simulink model "momentumBasedFlight"  (Simulink 10.3)
settings: Solver=FixedStepAuto  StartTime=0.0  StopTime=Config.simulationTime  FixedStep=Config.tStep  RelTol=1e-3
InitFcn:
  | cd(fileparts(which(bdroot)));
  | initMomentumBasedFlight;
StopFcn:
  | cd(fileparts(which(bdroot)));
  | stopMomentumBasedFlight;
undefined symbols (not defined in the file or in its folder): biasVectorConstraint_feet, Config, confVisualizer, ConstraintMatrix_feet, DiscIntNeverNeededParam, jets_config
undefined symbols (not defined in the file): Frames
libraries: WBToolboxLibrary x25, momentum_flight_control_sublib x2, thrust_estimation_sublib x1, jets_control x1, iDynVisualizer x1
(part 3 of 3)

== matlab function FLIGHT CONTROLLER (CORE) V2.5 - AERO/Flight Controller RAL-HUMANOIDS V3.0 - AERODYNAMICS/Joint Torque Control for Flying/torqueControlFCN ==
  data: M input double; h input double; J_jets input double; J_LFoot input double; J_RFoot input double; JDot_LFoot_nu input double; JDot_RFoot_nu input double; J_com input double; w_H_LFoot input double; w_H_RFoot input double; matrixOfJetsAxes input double; ConstraintsMatrix_feet input double; biasVectorConstraint_feet input double; jetsIntensities input double; stateVel input double; jointVel_star input double; contactForces_star input double; KI_torqueControl input double; KP_torqueControl input double; feetContactIsActive input double; activateEqConstrTorqueControl input double; robotIsLanded input double; jointPos_err input double; aerodynamic_force input double; Hessian output double; Config parameter double; gradient output double; ConstraintMatrix_inequality output double; biasVectorConstraint_inequality output double; jointVel_err output double
function [Hessian, gradient, ConstraintMatrix_inequality, biasVectorConstraint_inequality, jointVel_err] =  ... 
             flightTorqueControlFCN(M, h, J_jets, J_LFoot, J_RFoot, JDot_LFoot_nu, JDot_RFoot_nu, J_com, w_H_LFoot, w_H_RFoot, matrixOfJetsAxes, ...
                                    ConstraintsMatrix_feet, biasVectorConstraint_feet, jetsIntensities, stateVel, jointVel_star, contactForces_star, ...
                                    KI_torqueControl, KP_torqueControl, feetContactIsActive, activateEqConstrTorqueControl, robotIsLanded, jointPos_err, aerodynamic_force, Config)
                                      
    [Hessian, gradient, ConstraintMatrix_inequality, biasVectorConstraint_inequality, jointVel_err] =  ... 
             flightTorqueControl(M, h, J_jets, J_LFoot, J_RFoot, JDot_LFoot_nu, JDot_RFoot_nu, J_com, w_H_LFoot, w_H_RFoot, matrixOfJetsAxes, ...
                                 ConstraintsMatrix_feet, biasVectorConstraint_feet, jetsIntensities, stateVel, jointVel_star, contactForces_star, ...
                                 KI_torqueControl, KP_torqueControl, feetContactIsActive, activateEqConstrTorqueControl, robotIsLanded, jointPos_err, aerodynamic_force, Config);           
end

== matlab function FLIGHT CONTROLLER (CORE) V2.5 - AERO/Flight State Machine/Compute Gains And References/Trajectory Generator/Detect Robot Movement Request From Joystick ==
  data: joyAxes input double; moveFront output double; moveLateral output double; moveUpDown output double; rotateRoll output double; rotatePitch output double; joyButtons input double; rotateYaw output double; turbo_mode output double; goLandingPos output double
function [moveFront,moveLateral,moveUpDown,rotateRoll,rotatePitch,rotateYaw,turbo_mode,goLandingPos] = detectMovementsFromJoystickFCN(joyAxes,joyButtons)

    [moveFront,moveLateral,moveUpDown,rotateRoll,rotatePitch,rotateYaw,turbo_mode,goLandingPos] = iRonCubLib.detectMovementsFromJoystick(joyAxes,joyButtons);
end

== matlab function FLIGHT CONTROLLER (CORE) V2.5 - AERO/Flight State Machine/Take Off//Landing State Detector/MATLAB Function ==
  data: wrench_l input double; feetContactIsActive output double; wrench_r input double; Config parameter double; robotIsLanded output double; oneFootIsInContact output double
function [feetContactIsActive, robotIsLanded, oneFootIsInContact] = feetContactActivationFCN(wrench_l, wrench_r, Config)

    [feetContactIsActive, robotIsLanded, oneFootIsInContact] = iRonCubLib.feetContactActivation(wrench_l, wrench_r, Config);
end

== matlab function FLIGHT CONTROLLER (CORE) V2.5 - AERO/Flight Controller RAL-HUMANOIDS V3.0 - AERODYNAMICS/Momentum Control for Flying/Momentum Control/Flying Controller Momentum FCN  ==
  data: jointPos input double; w_baseTwist input double; jetsIntensities input double; J_jets input double; J_CoM input double; J_LFoot input double; J_RFoot input double; posCoM input double; w_R_b input double; w_H_LFoot input double; w_H_RFoot input double; matrixOfJetsAxes input double; matrixOfJetsArms input double; w_I_c input double; L input double; M input double; CMM input double; pos_vel_acc_jerk_CoM_des input double; rot_vel_acc_jerk_base_des input double size=[3,6]; jointPos_des input double; KP_momentum input double; KD_momentum input double; KP_postural input double; feetContactIsActive input double; decreaseMaxFootVerticalForce input double; increaseMinFootVerticalForce input double; robotIsLanded input double; HessianMatrixQP output double; gVectorQP output double; lowerBoundQP output double; upperBoundQP output double; L_des output double; LDot_estimated output double; verifyAngMomAndInertia output double; contactForces_hat input double; aerodynamic_force input double; Config parameter double
function [HessianMatrixQP, gVectorQP, lowerBoundQP, upperBoundQP, L_des, LDot_estimated, verifyAngMomAndInertia] = ...
             flightMomentumControlFCN(jointPos, w_baseTwist, jetsIntensities, J_jets, J_CoM, J_LFoot, J_RFoot, posCoM, w_R_b, w_H_LFoot, ...
                                      w_H_RFoot, matrixOfJetsAxes, matrixOfJetsArms, w_I_c, L, M, CMM, pos_vel_acc_jerk_CoM_des, ....
                                      rot_vel_acc_jerk_base_des, jointPos_des, KP_momentum, KD_momentum, KP_postural, feetContactIsActive, ...
                                      decreaseMaxFootVerticalForce, increaseMinFootVerticalForce, robotIsLanded, contactForces_hat, aerodynamic_force, Config)
                               
    [HessianMatrixQP, gVectorQP, lowerBoundQP, upperBoundQP, L_des, LDot_estimated, verifyAngMomAndInertia] = ...
             flightMomentumControl(jointPos, w_baseTwist, jetsIntensities, J_jets, J_CoM, J_LFoot, J_RFoot, posCoM, w_R_b, w_H_LFoot, ...
                                   w_H_RFoot, matrixOfJetsAxes, matrixOfJetsArms, w_I_c, L, M, CMM, pos_vel_acc_jerk_CoM_des, ....
                                   rot_vel_acc_jerk_base_des, jointPos_des, KP_momentum, KD_momentum, KP_postural, feetContactIsActive, ...
                                   decreaseMaxFootVerticalForce, increaseMinFootVerticalForce, robotIsLanded, contactForces_hat, aerodynamic_force, Config);
end

== matlab function FLIGHT CONTROLLER (CORE) V2.5 - AERO/Flight State Machine/Take Off//Landing State Detector/Vertical Forces Control ==
  data: joyButtons input double; decreaseMaxFootVerticalForce output double; increaseMinFootVerticalForce output double; activateEqConstrTorqueControl output double
function [decreaseMaxFootVerticalForce, increaseMinFootVerticalForce, activateEqConstrTorqueControl] = verticalForcesControlFCN(joyButtons)

    [decreaseMaxFootVerticalForce, increaseMinFootVerticalForce, activateEqConstrTorqueControl] = iRonCubLib.verticalForcesControl(joyButtons);
end

== matlab function FLIGHT CONTROLLER (CORE) V2.5 - AERO/Flight Controller RAL-HUMANOIDS V3.0 - AERODYNAMICS/Momentum Control for Flying/QP Solver and Integrate Contact Forces Derivative/Integrate the Contact Forces Derivative/deadZone/Deadzone Function ==
  data: u input double; y output double; thr input double
function y = deadZoneFCN(u, thr)

    y = wbc.deadZone(u, thr);
end

== matlab function Wind Generator/MATLAB Function ==
  data: t input double; v_wind output double; Config parameter double
function v_wind= generate_windFCN(t, Config)

v_wind = generate_wind(t,Config);

end

== matlab function FLIGHT CONTROLLER (CORE) V2.5 - AERO/Flight State Machine/Compute Gains And References/High-speed Flight Trajectory Generator/Trajectory Design for High Speed Motion  ==
  data: t input double; pos_vel_acc_jerk_CoM_des output double; posCoM_init input double; turbo_mode_hs output double; Config parameter double
function [pos_vel_acc_jerk_CoM_des, turbo_mode_hs] = high_speed_trajectory_designFCN(t, posCoM_init, Config)

[pos_vel_acc_jerk_CoM_des, turbo_mode_hs] = high_speed_trajectory_design(t, posCoM_init, Config);

end

== matlab function FLIGHT CONTROLLER (CORE) V2.5 - AERO/Flight Controller RAL-HUMANOIDS V3.0 - AERODYNAMICS/Momentum Control for Flying/QP Solver and Integrate Contact Forces Derivative/QP momentumControl/Process QP Inputs Momentum Control ==
  data: HessianMatrixQP input double; H_balancing output double; gVectorQP input double; lowerBoundQP input double; upperBoundQP input double; g_balancing output double; ub_balancing output double; lb_balancing output double; H_flight output double; g_flight output double; ub_flight output double; lb_flight output double
function [H_balancing,g_balancing,ub_balancing,lb_balancing, ...
          H_flight,g_flight,ub_flight,lb_flight] = processQPinputMomentumControlFCN(HessianMatrixQP,gVectorQP,lowerBoundQP,upperBoundQP) 
      
    [H_balancing,g_balancing,ub_balancing,lb_balancing, ...
        H_flight,g_flight,ub_flight,lb_flight] = iRonCubLib.processQPinputMomentumControl(HessianMatrixQP,gVectorQP,lowerBoundQP,upperBoundQP);
end

== matlab function FLIGHT CONTROLLER (CORE) V2.5 - AERO/Get System State/Change Contact Forces Representation/Change Contact Forces Representation ==
  data: contactForces_WBD input double; mixed_f_l_sole output double; w_R_l_sole input double; w_R_r_sole input double; mixed_f_r_sole output double
function [mixed_f_l_sole,mixed_f_r_sole] = fromBodyFrameToMixed_contactForcesFCN(contactForces_WBD,w_R_l_sole,w_R_r_sole)

    [mixed_f_l_sole,mixed_f_r_sole] = iRonCubLib.fromBodyFrameToMixed_contactForces(contactForces_WBD,w_R_l_sole,w_R_r_sole);
end

== matlab function FLIGHT CONTROLLER (CORE) V2.5 - AERO/Flight State Machine/Compute Gains And References/Compute Gains/Apply Gain Scheduling on Momentum Gains ==
  data: posCoM input double; KP_momentum_vector output double; posCoM_des input double; KD_momentum_vector output double; Config parameter double
function [KP_momentum_vector, KD_momentum_vector] = gain_scheduling_linear_momentumFCN(posCoM, posCoM_des, Config)

[KP_momentum_vector, KD_momentum_vector] = gain_scheduling_linear_momentum(posCoM, posCoM_des, Config);
end

== matlab function FLIGHT CONTROLLER (CORE) V2.5 - AERO/Flight Controller RAL-HUMANOIDS V3.0 - AERODYNAMICS/Momentum Control for Flying/QP Solver and Integrate Contact Forces Derivative/Integrate the Contact Forces Derivative/Select Integrator Initial Condition ==
  data: feetContactIsActive input double; contactForces input double; contactForces_0 output double
function contactForces_0 = selectInitContactForcesFCN(feetContactIsActive, contactForces)

    contactForces_0 = iRonCubLib.selectInitContactForces(feetContactIsActive, contactForces);
end

== matlab function FLIGHT CONTROLLER (CORE) V2.5 - AERO/Flight State Machine/Compute Gains And References/Smooth CoM and Base References/Smooth Reference Orientations/Rotational PID Controller/Compute Rotation Matrix Derivative ==
  data: gainSmoothingBaseRot input double; w_R_b_des input double; w_R_b input double; b_omega_b output double; RDot output double
function [b_omega_b, RDot] = rotationDerivativeFromAngVelFCN(gainSmoothingBaseRot, w_R_b_des, w_R_b)
                                                                                                                                                            
    % Rotational PID: 
    %
    % w_R_b_des = reference rotation (may be discontinuous)
    % 
    % b_omega_b = control input for the rotational PID. The angular velocity
    %             is expressed w.r.t. a frame attached to the link, i.e. it 
    %             is expressed in the "body" frame (b).
    % 
    % Kp        = control gain
    %
    % w_R_b     = smooth base rotation
    %
    b_omega_b_des       = zeros(3,1);
    Kp                  = gainSmoothingBaseRot;
    b_omega_b           = wbc.rotationalPID_bodyVelocity(w_R_b, w_R_b_des, b_omega_b_des, Kp);
                      
    % compute the rotation matrix derivative given the angular velocity in body frame
    RDot                = wbc.rotationDerivativeFromBodyAngVel(b_omega_b, w_R_b); 
end
